simulink model "proj3_oldest"  (R2021a)
settings: Solver=VariableStepAuto  StartTime=0.0  StopTime=30  RelTol=1e-3
libraries: hdlBasic x40, xbsIndex_r4 x1
settings Model: Creator=jag33  LastModifiedBy=jag33

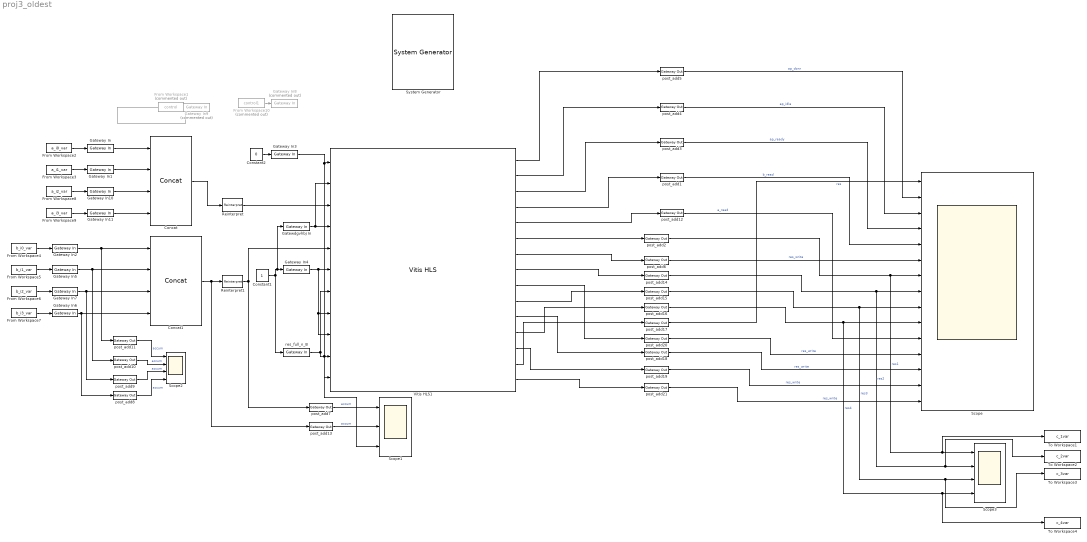
== system proj3_oldest ==
  " System Generator" : xbsIndex_r4/ System Generator  Tag=genX  xilinxfamily=zynq  part=xc7z020  speed=-1  package=clg484  synthesis_tool=Vivado  clock_wrapper=Clock Enables  directory=./netlist_proj3  proj_type=Vivado  Synth_file=Vivado Synthesis Defaults  Impl_file=Vivado Implementation Defaults  testbench=off  simulink_period=1  sysclk_period=10  dcm_input_clock_period=10  incr_netlist=off  trim_vbits=Everywhere in SubSystem  dbl_ovrd=According to Block Masks  core_generation=According to Block Masks  run_coregen=off  deprecated_control=off  eval_field=0  block_type=sysgen
  Concat : hdlBasic/Concat  num_inputs=4  XmcBlockStatus=1  maskContainerNames=group1  block_type=concat  block_config=sysgen:Concat_config
  Concat1 : hdlBasic/Concat  num_inputs=4  XmcBlockStatus=1  maskContainerNames=group1  block_type=concat  block_config=sysgen:Concat_config
  Constant1 : Constant
  Constant2 : Constant  Value=0
  From Workspace1 : FromWorkspace  Commented=on  VariableName=control
  From Workspace10 : FromWorkspace  Commented=on  VariableName=control1
  From Workspace2 : FromWorkspace  VariableName=a_i0_var
  From Workspace3 : FromWorkspace  VariableName=a_i1_var
  From Workspace4 : FromWorkspace  VariableName=b_i0_var
  From Workspace5 : FromWorkspace  VariableName=b_i1_var
  From Workspace6 : FromWorkspace  VariableName=b_i2_var
  From Workspace7 : FromWorkspace  VariableName=b_i3_var
  From Workspace8 : FromWorkspace  VariableName=a_i2_var
  From Workspace9 : FromWorkspace  VariableName=a_i3_var
  Gateway In{,1..2,5..7,10..11} (8 alike) : hdlBasic/Gateway In  gui_display_data_type=Fixed-point  arith_type=Unsigned  n_bits=16  bin_pt=0  preci_type=Single  exp_width=8  frac_width=24  rows=1  columns=1  quantization="Round  (unbiased: +/- Inf)"  overflow=Saturate  period=1  UseAsADC=off  ADCChannel='1'  interface=None  automatic_assignment=on  address_offset=hex2dec('00')  intf_name=''  intf_description=''  default_value=0  timing_constraint=None  locs_specified=off  LOCs={}  io_standard={}  inherit_from_input=off  hdl_port=on  XmcBlockStatus=1  maskContainerNames=group4  block_type=gatewayin  block_config=sysgen:gateway_in_config  block_width_w=590  block_height_w=620  block_width=640  block_height=850
  Gateway In3 : hdlBasic/Gateway In  gui_display_data_type=Boolean  arith_type=Boolean  n_bits=16  bin_pt=0  preci_type=Single  exp_width=8  frac_width=24  rows=1  columns=1  quantization="Round  (unbiased: +/- Inf)"  overflow=Saturate  period=1  UseAsADC=off  ADCChannel='1'  interface=None  automatic_assignment=on  address_offset=hex2dec('00')  intf_name=''  intf_description=''  default_value=0  timing_constraint=None  locs_specified=off  LOCs={}  io_standard={}  inherit_from_input=off  hdl_port=on  XmcBlockStatus=1  maskContainerNames=group4  block_type=gatewayin  block_config=sysgen:gateway_in_config  block_width_w=590  block_height_w=620  block_width=640  block_height=850
  Gateway In4 : hdlBasic/Gateway In  gui_display_data_type=Boolean  arith_type=Boolean  n_bits=16  bin_pt=0  preci_type=Single  exp_width=8  frac_width=24  rows=1  columns=1  quantization="Round  (unbiased: +/- Inf)"  overflow=Saturate  period=1  UseAsADC=off  ADCChannel='1'  interface=None  automatic_assignment=on  address_offset=hex2dec('00')  intf_name=''  intf_description=''  default_value=0  timing_constraint=None  locs_specified=off  LOCs={}  io_standard={}  inherit_from_input=off  hdl_port=on  XmcBlockStatus=1  maskContainerNames=group4  block_type=gatewayin  block_config=sysgen:gateway_in_config  block_width_w=590  block_height_w=620  block_width=640  block_height=850
  Gateway In8 : hdlBasic/Gateway In  Commented=on  gui_display_data_type=Boolean  arith_type=Boolean  n_bits=16  bin_pt=0  preci_type=Single  exp_width=8  frac_width=24  rows=1  columns=1  quantization="Round  (unbiased: +/- Inf)"  overflow=Saturate  period=1  UseAsADC=off  ADCChannel='1'  interface=None  automatic_assignment=on  address_offset=hex2dec('00')  intf_name=''  intf_description=''  default_value=0  timing_constraint=None  locs_specified=off  LOCs={}  io_standard={}  inherit_from_input=off  hdl_port=on  XmcBlockStatus=1  maskContainerNames=group4  block_type=gatewayin  block_config=sysgen:gateway_in_config  block_width_w=590  block_height_w=620  block_width=640  block_height=850
  Gateway In9 : hdlBasic/Gateway In  Commented=on  gui_display_data_type=Boolean  arith_type=Boolean  n_bits=16  bin_pt=0  preci_type=Single  exp_width=8  frac_width=24  rows=1  columns=1  quantization="Round  (unbiased: +/- Inf)"  overflow=Saturate  period=1  UseAsADC=off  ADCChannel='1'  interface=None  automatic_assignment=on  address_offset=hex2dec('00')  intf_name=''  intf_description=''  default_value=0  timing_constraint=None  locs_specified=off  LOCs={}  io_standard={}  inherit_from_input=off  hdl_port=on  XmcBlockStatus=1  maskContainerNames=group4  block_type=gatewayin  block_config=sysgen:gateway_in_config  block_width_w=590  block_height_w=620  block_width=640  block_height=850
  Gatewdgvhbj In : hdlBasic/Gateway In  gui_display_data_type=Boolean  arith_type=Boolean  n_bits=16  bin_pt=14  preci_type=Single  exp_width=8  frac_width=24  rows=1  columns=1  quantization="Round  (unbiased: +/- Inf)"  overflow=Saturate  period=1  UseAsADC=off  ADCChannel='1'  interface=None  automatic_assignment=on  address_offset=hex2dec('00')  intf_name=''  intf_description=''  default_value=0  timing_constraint=None  locs_specified=off  LOCs={}  io_standard={}  inherit_from_input=off  hdl_port=on  XmcBlockStatus=1  maskContainerNames=group4  block_type=gatewayin  block_config=sysgen:gateway_in_config  block_width_w=590  block_height_w=620  block_width=640  block_height=850
  Reinterpret : hdlBasic/Reinterpret  force_arith_type=on  arith_type="Signed  (2's comp)"  force_bin_pt=off  bin_pt=0  XmcBlockStatus=1  maskContainerNames=group1  block_type=reinterpret  block_config=sysgen:Reinterpret_config
  Reinterpret1 : hdlBasic/Reinterpret  force_arith_type=on  arith_type="Signed  (2's comp)"  force_bin_pt=off  bin_pt=0  XmcBlockStatus=1  maskContainerNames=group1  block_type=reinterpret  block_config=sysgen:Reinterpret_config
  Scope : Scope  NumInputPorts=15
  Scope1 : Scope  NumInputPorts=3
  Scope2 : Scope  NumInputPorts=4
  Scope3 : Scope  NumInputPorts=4
  To Workspace1 : ToWorkspace  VariableName=c_1var  SaveFormat=Timeseries  SampleTime=-1
  To Workspace2 : ToWorkspace  VariableName=c_2var  SaveFormat=Timeseries  SampleTime=-1
  To Workspace3 : ToWorkspace  VariableName=c_3var  SaveFormat=Timeseries  SampleTime=-1
  To Workspace4 : ToWorkspace  VariableName=c_4var  SaveFormat=Timeseries  SampleTime=-1
  Vitis HLS1 : hdlBasic/Vitis HLS  anytable='.\solution1\solution1'  fast_sim=off  display_datatype=on  rate_propagation_method=Simulink system period  model_file_path=''  latency=1  block_type=vitis_hls
      settings: infoedit=This block allows including C,C++ and SystemC source files in System Generator for DSP designs.
  post_add{1..6,12,14..21} (15 alike) : hdlBasic/Gateway Out  inherit_from_input=off  hdl_port=on  rows=1  columns=1  UseAsDAC=off  DACChannel='1'  interface=None  automatic_assignment=on  address_offset=hex2dec('00')  intf_name=''  intf_description=''  timing_constraint=None  locs_specified=off  LOCs={}  io_standard={}  XmcBlockStatus=1  maskContainerNames=group4  block_type=gatewayout  block_config=sysgen:gateway_out_config  block_width_w=590  block_height_w=620  block_width=620  block_height=750
  post_add{7..11,13} (6 alike) : hdlBasic/Gateway Out  inherit_from_input=on  hdl_port=on  rows=1  columns=1  UseAsDAC=off  DACChannel='1'  interface=None  automatic_assignment=on  address_offset=hex2dec('00')  intf_name=''  intf_description=''  timing_constraint=None  locs_specified=off  LOCs={}  io_standard={}  XmcBlockStatus=1  maskContainerNames=group4  block_type=gatewayout  block_config=sysgen:gateway_out_config  block_width_w=590  block_height_w=620  block_width=620  block_height=750
  res_full_n_B : hdlBasic/Gateway In  gui_display_data_type=Boolean  arith_type=Boolean  n_bits=16  bin_pt=0  preci_type=Single  exp_width=8  frac_width=24  rows=1  columns=1  quantization="Round  (unbiased: +/- Inf)"  overflow=Saturate  period=1  UseAsADC=off  ADCChannel='1'  interface=None  automatic_assignment=on  address_offset=hex2dec('00')  intf_name=''  intf_description=''  default_value=0  timing_constraint=None  locs_specified=off  LOCs={}  io_standard={}  inherit_from_input=off  hdl_port=on  XmcBlockStatus=1  maskContainerNames=group4  block_type=gatewayin  block_config=sysgen:gateway_in_config  block_width_w=590  block_height_w=620  block_width=640  block_height=850
  wires:
  From Workspace1/1 -> Gateway In9/1
  res_full_n_B/1 -> Vitis HLS1/11, Vitis HLS1/10, Vitis HLS1/7
  Vitis HLS1/6 -> post_add2/1
  Vitis HLS1/7 -> post_add6/1
  Vitis HLS1/4 -> post_add1/1
  Vitis HLS1/3 -> post_add3/1
  Vitis HLS1/2 -> post_add4/1
  Vitis HLS1/1 -> post_add5/1
  post_add5/1 -> Scope/2  "ap_donr"
  post_add4/1 -> Scope/3  "ap_idle"
  post_add3/1 -> Scope/4  "ap_ready"
  post_add1/1 -> Scope/5  "b_read"
  Gateway In4/1 -> Vitis HLS1/9, Vitis HLS1/8, Vitis HLS1/6
  Reinterpret/1 -> Vitis HLS1/3
  Gatewdgvhbj In/1 -> Vitis HLS1/2, Vitis HLS1/4
  Reinterpret1/1 -> Vitis HLS1/5, post_add7/1
  Vitis HLS1/5 -> post_add12/1
  From Workspace5/1 -> Gateway In5/1
  From Workspace8/1 -> Gateway In10/1
  From Workspace4/1 -> Gateway In2/1
  From Workspace9/1 -> Gateway In11/1
  From Workspace3/1 -> Gateway In1/1
  From Workspace2/1 -> Gateway In/1
  Gateway In2/1 -> post_add11/1, Concat1/1
  Gateway In5/1 -> Concat1/2, post_add10/1
  Gateway In7/1 -> post_add9/1, Concat1/3
  Gateway In6/1 -> post_add8/1, Concat1/4
  Concat1/1 -> post_add13/1, Reinterpret1/1
  Gateway In/1 -> Concat/1
  Gateway In1/1 -> Concat/2
  Gateway In10/1 -> Concat/3
  Concat/1 -> Reinterpret/1
  Gateway In11/1 -> Concat/4
  post_add7/1 -> Scope1/1  "accum"
  From Workspace6/1 -> Gateway In7/1
  From Workspace7/1 -> Gateway In6/1
  post_add8/1 -> Scope2/4  "accum"
  post_add11/1 -> Scope2/1  "accum"
  post_add10/1 -> Scope2/2  "accum"
  post_add9/1 -> Scope2/3  "accum"
  post_add13/1 -> Scope1/2  "accum"
  Constant1/1 -> res_full_n_B/1, Gatewdgvhbj In/1, Gateway In4/1
  post_add14/1 -> Scope/8, To Workspace2/1, Scope3/2  "res2"
  post_add15/1 -> Scope/9, To Workspace3/1, Scope3/3  "res3"
  post_add16/1 -> Scope/10, To Workspace4/1, Scope3/4  "res4"
  post_add19/1 -> Scope/14  "res_write"
  post_add18/1 -> Scope/13  "res_write"
  post_add17/1 -> Scope/1  "res"
  post_add21/1 -> Scope/15  "res_write"
  post_add20/1 -> Scope/12  "res_write"
  Vitis HLS1/8 -> post_add14/1
  Vitis HLS1/10 -> post_add15/1
  Vitis HLS1/9 -> post_add20/1
  Vitis HLS1/11 -> post_add18/1
  Vitis HLS1/13 -> post_add19/1
  post_add12/1 -> Scope/11  "a_read"
  post_add6/1 -> Scope/6  "res_write"
  post_add2/1 -> Scope/7, To Workspace1/1, Scope3/1  "res1"
  Vitis HLS1/12 -> post_add16/1
  Gateway In3/1 -> Scope1/3, Vitis HLS1/1
  Constant2/1 -> Gateway In3/1
  From Workspace10/1 -> Gateway In8/1
  Vitis HLS1/14 -> post_add17/1
  Vitis HLS1/15 -> post_add21/1
